simulink model "pwm"  (R2014b)
settings: Solver=ode45  StartTime=0.0  StopTime=1/100  RelTol=1e-3
model workspace (MAT data in the model file):
  amplitude = Simulink.Parameter
  amplitude.Value = 1
  amplitude.DataType = 'auto'
  freqency = Simulink.Parameter
  freqency.Value = 10000
  freqency.DataType = 'auto'
libraries: simulink x1
settings Model: Creator=sbrooks  LastModifiedBy=sbrooks

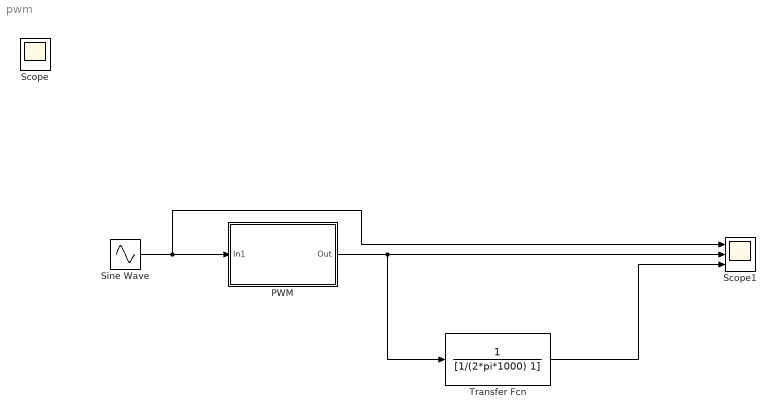
== system pwm ==
  PWM : Subsystem  mask(Ideal PWM Generator){amplitude=1, frequency=100000}
      mask help: Generates a 0-[Amplitude] output PWM signal at [Frequency] modulation frequency.
  Scope1 : Scope  NumInputPorts=3
      settings: YMin=-5~-5~-5  YMax=5~5~5
  Sine Wave : Sin  Frequency=1000*2*pi  SampleTime=0
  Transfer Fcn : TransferFcn  Denominator=[1/(2*pi*1000) 1]
  Scope : Scope
  wires:
  Sine Wave/1 -> Scope1/1, PWM/1(In1)
  PWM/1(Out) -> Scope1/2, Transfer Fcn/1
  Transfer Fcn/1 -> Scope1/3

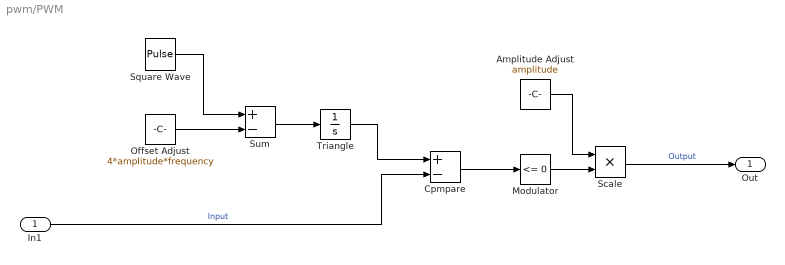
== system pwm/PWM ==
  In1 : Inport
  Amplitude Adjust : Constant  Value=amplitude
  Cpmpare : Sum  Inputs=+-
  Modulator : simulink/Logic and Bit Operations/Compare To Zero  relop=<=  OutDataTypeStr=boolean
  Offset Adjust : Constant  Value=4*amplitude*frequency
  Scale : Product
  Square Wave : DiscretePulseGenerator  PulseType=Time based  Amplitude=8*amplitude*frequency  Period=1/frequency  PulseWidth=50  PhaseDelay=-1/(frequency*4)
  Sum : Sum  Inputs=+-
  Triangle : Integrator
  Out : Outport
  wires:
  Triangle/1 -> Cpmpare/1
  In1/1 -> Cpmpare/2  "Input"
  Offset Adjust/1 -> Sum/2
  Sum/1 -> Triangle/1
  Square Wave/1 -> Sum/1
  Scale/1 -> Out/1  "Output"
  Amplitude Adjust/1 -> Scale/1
  Modulator/1 -> Scale/2
  Cpmpare/1 -> Modulator/1
